simulink model "martins_version_wconv"  (R2023b)
settings: Solver=VariableStepAuto  StartTime=0.0  StopTime=Tend  RelTol=1e-3
undefined symbols (not defined in the file): C_dc, c_f, C_hv_km, Cagg, DiscIntNeverNeededParam, H_vsm, Ibase_hv, Ibase_lv, Ibase_mv, k_AD, k_d_vsm, k_decouple, k_ffv, k_ic, k_idc, k_mod, k_p_p_vsm, k_p_q_vsm, k_pc, k_pdc, k_vc, KG_LL, ki, KI_LL, ki_q, kp, KP_LL, kslope_VSC, L_comp, l_f, l_f_si1, l_grid, L_hv_km, l_t_ehvhv, l_t_hvmv, l_t_mvlv, L_Virt, Lagg, Lbase1v, length_export, omega_nom, P_aero_0, phase_shift_test_state, phase_shifts, pie_export, r_f, r_f_si1, r_grid, R_hv_km, r_t_ehvhv, r_t_hvmv, r_t_mvlv, R_Virt, Ragg, rocof_slope, Rocof_test_state, Sbase1, Tchange_gfm_ref, Tdelay, Trocof_end ... (+13)
libraries: slpidlib x11, spsFirstOrderFilterLib x3, cstblocks x1, simulink x1, spsSampleandHoldLib x1, spspowerguiLib x1
(part 3 of 3)

== system martins_version_wconv/GFC_WT/grid>>PLL2 ==
  note: *
  note: =
  note: inv ([  cos(wt)   sin(wt)
      |    -sin(wt)    cos(wt)   ])
  note: [ d
      |    q ]
  note: [  al
      |     be  ]
  note: *
  note: =
  note: [  cos(wt)   -sin(wt)
      |    sin(wt)    cos(wt)   ]
  note: [ d
      |    q ]
  note: [  al
      |     be  ]
  vgDQ : Inport
  wt : Inport  Port=2
  Cos : Trigonometry  Operator=cos
  Demux1 : Demux  Outputs=2
  Display5 : Display
  Mux3 : Mux  Inputs=2
  Product{,1..3} (4 alike) : Product
  Sin : Trigonometry
  Sum : Sum
  Sum1 : Sum  Inputs=+-
  vgdq : Outport  InitialOutput=[0,0]  VectorParamsAs1DForOutWhenUnconnected=off
  wires:
  Demux1/1 -> Product/1, Product3/1
  wt/1 -> Sin/1, Cos/1
  Product/1 -> Sum/1
  Sum/1 -> Mux3/1
  Mux3/1 -> Display5/1, vgdq/1
  Sum1/1 -> Mux3/2
  vgDQ/1 -> Demux1/1
  Sin/1 -> Product1/2, Product3/2
  Product1/1 -> Sum/2
  Cos/1 -> Product/2, Product2/2
  Product2/1 -> Sum1/1
  Demux1/2 -> Product1/1, Product2/1
  Product3/1 -> Sum1/2

== system martins_version_wconv/GFC_WT/grid>>PLL3 ==
  note: *
  note: =
  note: inv ([  cos(wt)   sin(wt)
      |    -sin(wt)    cos(wt)   ])
  note: [ d
      |    q ]
  note: [  al
      |     be  ]
  note: *
  note: =
  note: [  cos(wt)   -sin(wt)
      |    sin(wt)    cos(wt)   ]
  note: [ d
      |    q ]
  note: [  al
      |     be  ]
  vgDQ : Inport
  wt : Inport  Port=2
  Cos : Trigonometry  Operator=cos
  Demux1 : Demux  Outputs=2
  Display5 : Display
  Mux3 : Mux  Inputs=[vect vect]
  Product{,1..3} (4 alike) : Product
  Sin : Trigonometry
  Sum : Sum
  Sum1 : Sum  Inputs=+-
  vgdq : Outport  InitialOutput=[0,0]  VectorParamsAs1DForOutWhenUnconnected=off
  wires:
  Demux1/1 -> Product/1, Product3/1
  wt/1 -> Sin/1, Cos/1
  Product/1 -> Sum/1
  Sum/1 -> Mux3/1
  Mux3/1 -> Display5/1, vgdq/1
  Sum1/1 -> Mux3/2
  vgDQ/1 -> Demux1/1
  Sin/1 -> Product1/2, Product3/2
  Product1/1 -> Sum/2
  Cos/1 -> Product/2, Product2/2
  Product2/1 -> Sum1/1
  Demux1/2 -> Product1/1, Product2/1
  Product3/1 -> Sum1/2

== system martins_version_wconv/GFC_WT/v_dc_reg ==
  In1 : Inport
  Ipart : DiscreteIntegrator  Commented=on  gainval=k_idc  SampleTime=-1  ICPrevOutput=DiscIntNeverNeededParam  ICPrevScaledInput=DiscIntNeverNeededParam
  PID Controller : slpidlib/PID Controller  Controller=PI  Form=Parallel  TimeDomain=Continuous-time  UseExternalTs=off  SampleTime=-1  IntegratorMethod=Forward Euler  FilterMethod=Forward Euler  ControllerParametersSource=internal  P=k_pdc  I=k_idc  UseKiTs=off  D=0  N=100  UseFilter=on  TunerSelectOption=Transfer Function Based (PID Tuner App)  InitialConditionSource=internal  InitialConditionForIntegrator=0  InitialConditionForFilter=0  DifferentiatorICPrevScaledInput=0  ExternalReset=none  TrackingMode=off  Kt=1  LimitOutput=off  SatLimitsSource=internal  UpperSaturationLimit=inf  LowerSaturationLimit=-inf  LinearizeAsGain=on  AntiWindupMode=none  Kb=1  LimitIntegrator=off  UpperIntegratorSaturationLimit=inf  LowerIntegratorSaturationLimit=-inf  POutMin=[]  POutMax=[]  IOutMin=[]  IOutMax=[]  DOutMin=[]  DOutMax=[]  NOutMin=[]  NOutMax=[]  SumOutMin=[]  SumOutMax=[]  SaturationOutMin=[]  SaturationOutMax=[]  PParamMin=[]  PParamMax=[]  IParamMin=[]  IParamMax=[]  DParamMin=[]  DParamMax=[]  NParamMin=[]  NParamMax=[]  KbParamMin=[]  KbParamMax=[]  KtParamMin=[]  KtParamMax=[]  KbOutMin=[]  KbOutMax=[]  KtOutMin=[]  KtOutMax=[]  IntegratorOutMin=[]  IntegratorOutMax=[]  FilterOutMin=[]  FilterOutMax=[]  SumI1OutMin=[]  SumI1OutMax=[]  SumI2OutMin=[]  SumI2OutMax=[]  SumI3OutMin=[]  SumI3OutMax=[]  SumI4OutMin=[]  SumI4OutMax=[]  SumDOutMin=[]  SumDOutMax=[]  DifferentiatorOutMin=[]  DifferentiatorOutMax=[]  FilterDiffOutCoefMin=[]  FilterDiffOutCoefMax=[]  ReciprocalOutMin=[]  ReciprocalOutMax=[]  SumDenOutMin=[]  SumDenOutMax=[]  SumNumOutMin=[]  SumNumOutMax=[]  DivideOutMin=[]  DivideOutMax=[]  UdiffTsProdOutMin=[]  UdiffTsProdOutMax=[]  NTsProdOutMin=[]  NTsProdOutMax=[]  UintegralTsProdOutMin=[]  UintegralTsProdOutMax=[]  UngainTsProdOutMin=[]  UngainTsProdOutMax=[]  ClampingZeroOutDataTypeStr=Inherit: Inherit via back propagation  ClampingZeroOutMin=[]  ClampingZeroOutMax=[]  FilterDenConstantOutDataTypeStr=Inherit: Inherit via back propagation  FilterDenConstantOutMin=[]  FilterDenConstantOutMax=[]  PCopyOutDataTypeStr=Inherit: Inherit via back propagation  PCopyOutMin=[]  PCopyOutMax=[]  NCopyOutDataTypeStr=Inherit: Inherit via back propagation  NCopyOutMin=[]  NCopyOutMax=[]  IntegratorContinuousStateAttributes=''  IntegratorStateMustResolveToSignalObject=off  IntegratorRTWStateStorageClass=Auto  FilterContinuousStateAttributes=''  FilterStateMustResolveToSignalObject=off  FilterRTWStateStorageClass=Auto  ParallelPVariant=InternalParameters  IdealPVariant=Disabled  IVariant=InternalParameters  DVariant=Disabled  IntegratorVariant=Continuous  SatVariant=Disabled  AWVariant=Passthrough  PCopyVariant=Disabled  TRVariant=Disabled  FdbkBlocksVariant=Forward  IdealPFdbkVariant=Disabled  SatFdbkVariant=Disabled  DerivativeFilterVariant=Disabled  NVariant=Disabled  NCopyVariant=Disabled_SignalSpec  FilterICVariant=Disabled  IntegratorICVariant=InternalICs  ExternalResetVariant=Disabled  TRSumVariant=Passthrough  SumFdbkVariant=Disabled  SumVariant=Sum_PI  TsampFilterVariant=InternalTs  TsampNgainVariant=Passthrough  TsampIntegralVariant=Disabled_SignalSpec  ExternalSaturationOutDataTypeStr=Inherit: Same as second input
  Ppart : Gain  Commented=on  Gain=k_pdc  SaturateOnIntegerOverflow=on  OutDataTypeStr=Inherit: Same as input  ParamDataTypeStr=Inherit: Same as input
  Sum5 : Sum  Commented=on  Inputs=|++  InputSameDT=on  SaturateOnIntegerOverflow=on  OutDataTypeStr=Inherit: Same as first input
  W : Outport
  wires:
  Ppart/1 -> Sum5/1
  Ipart/1 -> Sum5/2
  In1/1 -> PID Controller/1, Ppart/1, Ipart/1
  PID Controller/1 -> W/1

== system martins_version_wconv/HVAC CABLE 10 PI SEGMENTS 1/RC sys1 ==
  note: Left shunt capacitor
  note: shunt capacitor
  Iload_DQ : Inport
  "Isource_DQ " : Inport  Port=2
  omega_ref : Inport  Port=3
  1 : Gain  Gain=Rd
  10 : Gain  Gain=inv_Csource
  2 : Gain  Gain=Rd
  8 : Gain  Gain=Csource
  9 : Gain  Gain=inv_Csource
  Demux2 : Demux  Outputs=2
  Demux3 : Demux  Outputs=2
  Display1 : Display
  Display6 : Display
  Mux1 : Mux  Inputs=2
  Mux2 : Mux  Inputs=2
  Product7 : Product
  Product8 : Product
  Sum1 : Sum  Inputs=|++
  Sum14 : Sum  Inputs=|+--
  Sum15 : Sum  Inputs=|++-
  Sum2 : Sum  Inputs=|++
  Sum3 : Sum  Inputs=|+-
  Sum4 : Sum  Inputs=|+-
  Vcd : Scope
  VcpdR_int : Integrator  InitialCondition=VD0  UpperSaturationLimit=50  LowerSaturationLimit=-1000
  VcpqR_int : Integrator  InitialCondition=VQ0  UpperSaturationLimit=50  LowerSaturationLimit=-1000
  Vcq : Scope
  VpccR_DQ : Outport  VectorParamsAs1DForOutWhenUnconnected=off
  wires:
  8/1 -> [wcs], Display1/1
  Mux1/1 -> VpccR_DQ/1
  Product8/1 -> Sum14/3
  Sum15/1 -> 9/1
  10/1 -> VcpqR_int/1
  Product7/1 -> Sum15/1
  VcpqR_int/1 -> Mux2/1, Sum2/1, Product7/2, Vcq/1
  [wcs] -> Product7/1, Product8/1
  Sum14/1 -> 10/1
  9/1 -> VcpdR_int/1
  omega_ref/1 -> 8/1
  Demux2/1 -> Sum4/1, Sum15/2
  Demux2/2 -> Sum3/1, Sum14/1
  Iload_DQ/1 -> Demux2/1
  "Isource_DQ "/1 -> Demux3/1
  Demux3/2 -> Sum3/2, Sum14/2
  Demux3/1 -> Sum4/2, Sum15/3
  VcpdR_int/1 -> Mux2/2, Product8/2, Sum1/1
  Sum1/1 -> Mux1/1
  Sum2/1 -> Mux1/2
  1/1 -> Sum2/2
  2/1 -> Sum1/2
  Mux2/1 -> Display6/1
  Sum3/1 -> 1/1
  Sum4/1 -> 2/1

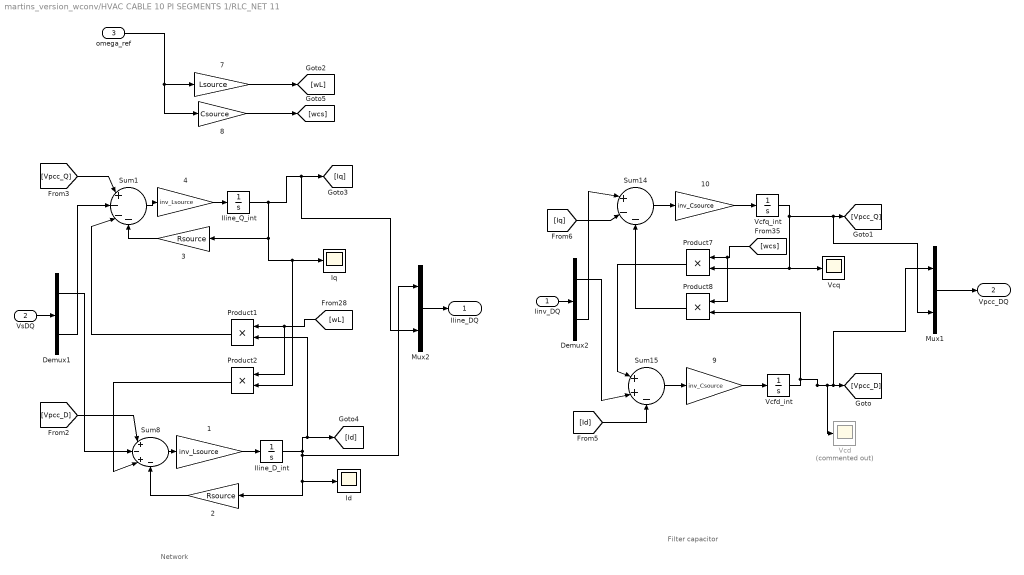
== system martins_version_wconv/HVAC CABLE 10 PI SEGMENTS 1/RLC_NET 11 ==
  note: Network
  note: Filter capacitor
  Iinv_DQ : Inport
  "VsDQ " : Inport  Port=2
  omega_ref : Inport  Port=3
  1 : Gain  Gain=inv_Lsource
  10 : Gain  Gain=inv_Csource
  2 : Gain  Gain=Rsource
  3 : Gain  Gain=Rsource
  4 : Gain  Gain=inv_Lsource
  7 : Gain  Gain=Lsource
  8 : Gain  Gain=Csource
  9 : Gain  Gain=inv_Csource
  Demux1 : Demux  Outputs=2
  Demux2 : Demux  Outputs=2
  Id : Scope
  Iline_D_int : Integrator  UpperSaturationLimit=50  LowerSaturationLimit=-1000
  Iline_Q_int : Integrator  UpperSaturationLimit=50  LowerSaturationLimit=-1000
  Iq : Scope
  Mux1 : Mux  Inputs=2
  Mux2 : Mux  Inputs=2
  Product{1..2,7..8} (4 alike) : Product
  Sum1 : Sum  Inputs=|+---
  Sum14 : Sum  Inputs=|+--
  Sum15 : Sum  Inputs=|++-
  Sum8 : Sum  Inputs=|+-+-
  Vcd : Scope  Commented=on
  Vcfd_int : Integrator  UpperSaturationLimit=50  LowerSaturationLimit=-1000
  Vcfq_int : Integrator  UpperSaturationLimit=50  LowerSaturationLimit=-1000
  Vcq : Scope
  Iline_DQ : Outport  VectorParamsAs1DForOutWhenUnconnected=off
  Vpcc_DQ : Outport  Port=2  VectorParamsAs1DForOutWhenUnconnected=off
  wires:
  Mux2/1 -> Iline_DQ/1
  Iinv_DQ/1 -> Demux2/1
  Demux2/2 -> Sum14/1
  Demux2/1 -> Sum15/2
  [wL] -> Product2/1, Product1/1
  Product1/1 -> Sum1/3
  4/1 -> Iline_Q_int/1
  3/1 -> Sum1/4
  Product2/1 -> Sum8/3
  2/1 -> Sum8/4
  Sum8/1 -> 1/1
  Iline_Q_int/1 -> 3/1, Product2/2, Iq/1, [Iq], Mux2/2
  Iline_D_int/1 -> Mux2/1, 2/1, Id/1, Product1/2, [Id]
  1/1 -> Iline_D_int/1
  Sum1/1 -> 4/1
  [Vpcc_D] -> Sum8/1
  [Vpcc_Q] -> Sum1/1
  omega_ref/1 -> 8/1, 7/1
  7/1 -> [wL]
  9/1 -> Vcfd_int/1
  Sum14/1 -> 10/1
  [wcs] -> Product8/1, Product7/1
  [Id] -> Sum15/3
  Vcfq_int/1 -> Mux1/2, [Vpcc_Q], Product7/2, Vcq/1
  Product7/1 -> Sum15/1
  [Iq] -> Sum14/2
  10/1 -> Vcfq_int/1
  Sum15/1 -> 9/1
  Product8/1 -> Sum14/3
  8/1 -> [wcs]
  Vcfd_int/1 -> Product8/2, Mux1/1, [Vpcc_D], Vcd/1
  Mux1/1 -> Vpcc_DQ/1
  Demux1/1 -> Sum8/2
  Demux1/2 -> Sum1/2
  "VsDQ "/1 -> Demux1/1

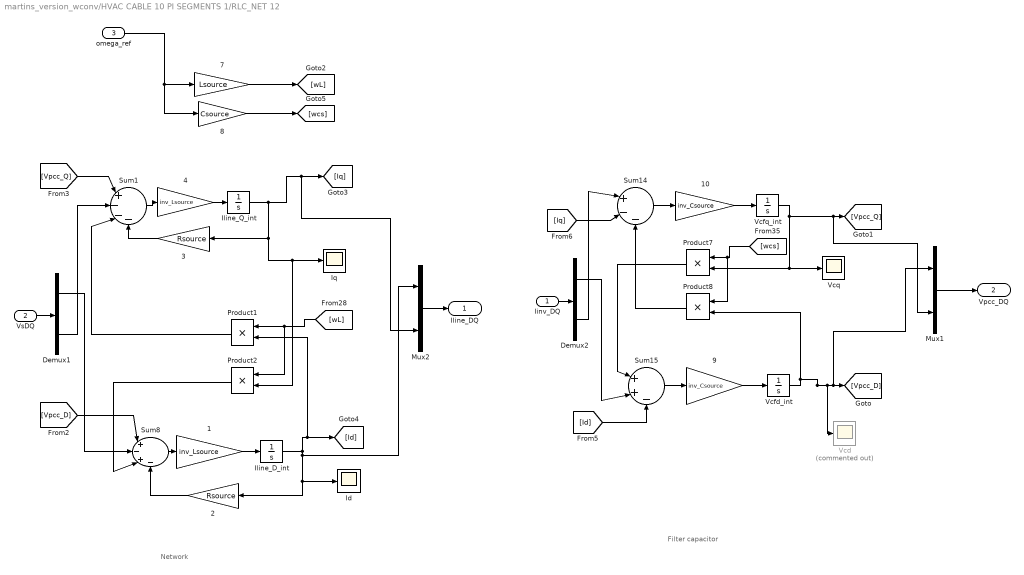
== system martins_version_wconv/HVAC CABLE 10 PI SEGMENTS 1/RLC_NET 12 ==
  note: Filter capacitor
  note: Network
  Iinv_DQ : Inport
  "VsDQ " : Inport  Port=2
  omega_ref : Inport  Port=3
  1 : Gain  Gain=inv_Lsource
  10 : Gain  Gain=inv_Csource
  2 : Gain  Gain=Rsource
  3 : Gain  Gain=Rsource
  4 : Gain  Gain=inv_Lsource
  7 : Gain  Gain=Lsource
  8 : Gain  Gain=Csource
  9 : Gain  Gain=inv_Csource
  Demux1 : Demux  Outputs=2
  Demux2 : Demux  Outputs=2
  Id : Scope
  Iline_D_int : Integrator  UpperSaturationLimit=50  LowerSaturationLimit=-1000
  Iline_Q_int : Integrator  UpperSaturationLimit=50  LowerSaturationLimit=-1000
  Iq : Scope
  Mux1 : Mux  Inputs=2
  Mux2 : Mux  Inputs=2
  Product{1..2,7..8} (4 alike) : Product
  Sum1 : Sum  Inputs=|+---
  Sum14 : Sum  Inputs=|+--
  Sum15 : Sum  Inputs=|++-
  Sum8 : Sum  Inputs=|+-+-
  Vcd : Scope  Commented=on
  Vcfd_int : Integrator  UpperSaturationLimit=50  LowerSaturationLimit=-1000
  Vcfq_int : Integrator  UpperSaturationLimit=50  LowerSaturationLimit=-1000
  Vcq : Scope
  Iline_DQ : Outport  VectorParamsAs1DForOutWhenUnconnected=off
  Vpcc_DQ : Outport  Port=2  VectorParamsAs1DForOutWhenUnconnected=off
  wires:
  "VsDQ "/1 -> Demux1/1
  Demux1/2 -> Sum1/2
  Demux1/1 -> Sum8/2
  Mux1/1 -> Vpcc_DQ/1
  Vcfd_int/1 -> Vcd/1, [Vpcc_D], Mux1/1, Product8/2
  8/1 -> [wcs]
  Product8/1 -> Sum14/3
  Sum15/1 -> 9/1
  10/1 -> Vcfq_int/1
  [Iq] -> Sum14/2
  Product7/1 -> Sum15/1
  Vcfq_int/1 -> Vcq/1, Product7/2, [Vpcc_Q], Mux1/2
  [Id] -> Sum15/3
  [wcs] -> Product7/1, Product8/1
  Sum14/1 -> 10/1
  9/1 -> Vcfd_int/1
  7/1 -> [wL]
  omega_ref/1 -> 7/1, 8/1
  [Vpcc_Q] -> Sum1/1
  [Vpcc_D] -> Sum8/1
  Sum1/1 -> 4/1
  1/1 -> Iline_D_int/1
  Iline_D_int/1 -> [Id], Product1/2, Id/1, 2/1, Mux2/1
  Iline_Q_int/1 -> Mux2/2, [Iq], Iq/1, Product2/2, 3/1
  Sum8/1 -> 1/1
  2/1 -> Sum8/4
  Product2/1 -> Sum8/3
  3/1 -> Sum1/4
  4/1 -> Iline_Q_int/1
  Product1/1 -> Sum1/3
  [wL] -> Product1/1, Product2/1
  Demux2/1 -> Sum15/2
  Demux2/2 -> Sum14/1
  Iinv_DQ/1 -> Demux2/1
  Mux2/1 -> Iline_DQ/1

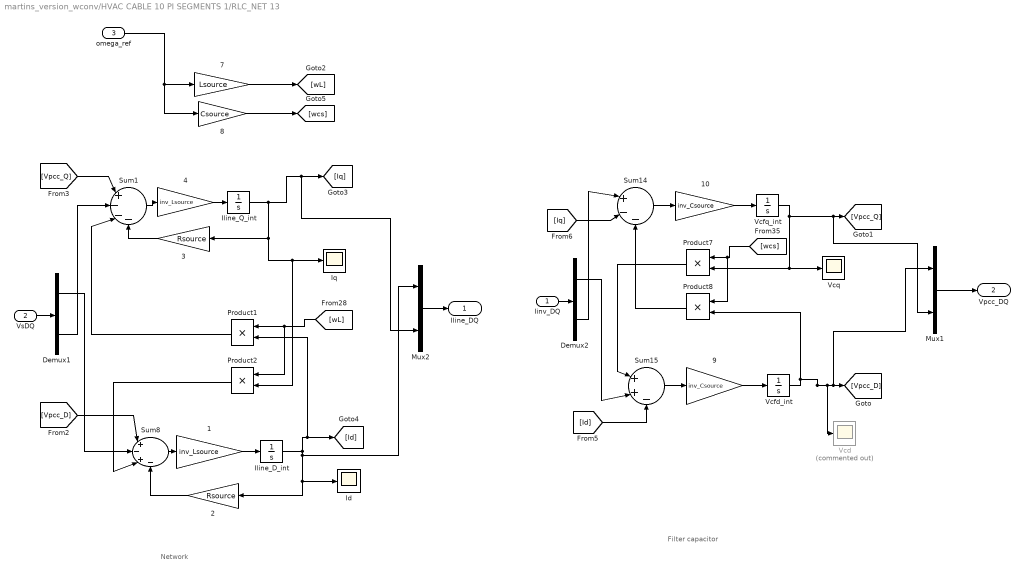
== system martins_version_wconv/HVAC CABLE 10 PI SEGMENTS 1/RLC_NET 13 ==
  note: Filter capacitor
  note: Network
  Iinv_DQ : Inport
  "VsDQ " : Inport  Port=2
  omega_ref : Inport  Port=3
  1 : Gain  Gain=inv_Lsource
  10 : Gain  Gain=inv_Csource
  2 : Gain  Gain=Rsource
  3 : Gain  Gain=Rsource
  4 : Gain  Gain=inv_Lsource
  7 : Gain  Gain=Lsource
  8 : Gain  Gain=Csource
  9 : Gain  Gain=inv_Csource
  Demux1 : Demux  Outputs=2
  Demux2 : Demux  Outputs=2
  Id : Scope
  Iline_D_int : Integrator  UpperSaturationLimit=50  LowerSaturationLimit=-1000
  Iline_Q_int : Integrator  UpperSaturationLimit=50  LowerSaturationLimit=-1000
  Iq : Scope
  Mux1 : Mux  Inputs=2
  Mux2 : Mux  Inputs=2
  Product{1..2,7..8} (4 alike) : Product
  Sum1 : Sum  Inputs=|+---
  Sum14 : Sum  Inputs=|+--
  Sum15 : Sum  Inputs=|++-
  Sum8 : Sum  Inputs=|+-+-
  Vcd : Scope  Commented=on
  Vcfd_int : Integrator  UpperSaturationLimit=50  LowerSaturationLimit=-1000
  Vcfq_int : Integrator  UpperSaturationLimit=50  LowerSaturationLimit=-1000
  Vcq : Scope
  Iline_DQ : Outport  VectorParamsAs1DForOutWhenUnconnected=off
  Vpcc_DQ : Outport  Port=2  VectorParamsAs1DForOutWhenUnconnected=off
  wires:
  "VsDQ "/1 -> Demux1/1
  Demux1/2 -> Sum1/2
  Demux1/1 -> Sum8/2
  Mux1/1 -> Vpcc_DQ/1
  Vcfd_int/1 -> Vcd/1, [Vpcc_D], Mux1/1, Product8/2
  8/1 -> [wcs]
  Product8/1 -> Sum14/3
  Sum15/1 -> 9/1
  10/1 -> Vcfq_int/1
  [Iq] -> Sum14/2
  Product7/1 -> Sum15/1
  Vcfq_int/1 -> Vcq/1, Product7/2, [Vpcc_Q], Mux1/2
  [Id] -> Sum15/3
  [wcs] -> Product7/1, Product8/1
  Sum14/1 -> 10/1
  9/1 -> Vcfd_int/1
  7/1 -> [wL]
  omega_ref/1 -> 7/1, 8/1
  [Vpcc_Q] -> Sum1/1
  [Vpcc_D] -> Sum8/1
  Sum1/1 -> 4/1
  1/1 -> Iline_D_int/1
  Iline_D_int/1 -> [Id], Product1/2, Id/1, 2/1, Mux2/1
  Iline_Q_int/1 -> Mux2/2, [Iq], Iq/1, Product2/2, 3/1
  Sum8/1 -> 1/1
  2/1 -> Sum8/4
  Product2/1 -> Sum8/3
  3/1 -> Sum1/4
  4/1 -> Iline_Q_int/1
  Product1/1 -> Sum1/3
  [wL] -> Product1/1, Product2/1
  Demux2/1 -> Sum15/2
  Demux2/2 -> Sum14/1
  Iinv_DQ/1 -> Demux2/1
  Mux2/1 -> Iline_DQ/1

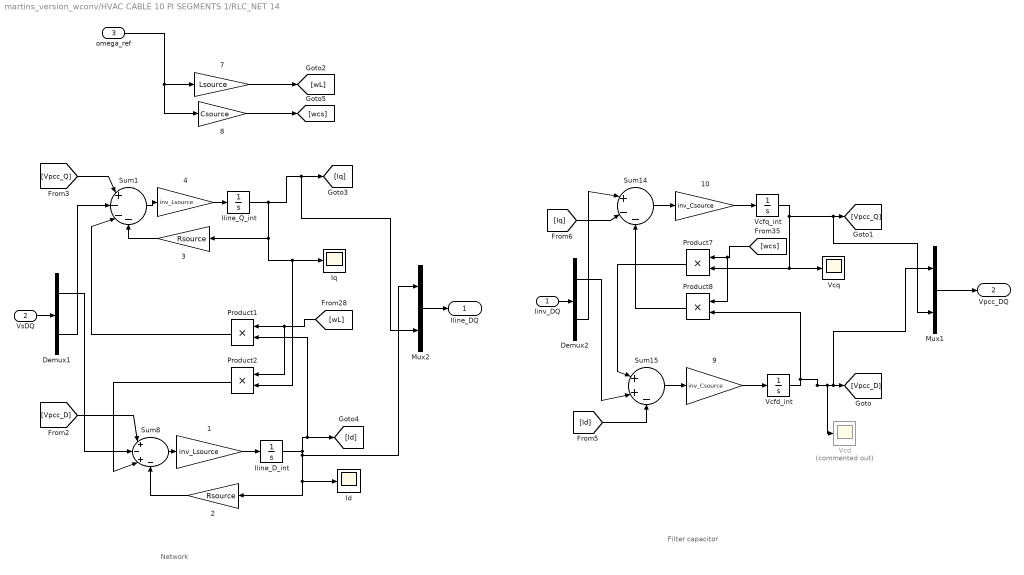
== system martins_version_wconv/HVAC CABLE 10 PI SEGMENTS 1/RLC_NET 14 ==
  note: Network
  note: Filter capacitor
  Iinv_DQ : Inport
  "VsDQ " : Inport  Port=2
  omega_ref : Inport  Port=3
  1 : Gain  Gain=inv_Lsource
  10 : Gain  Gain=inv_Csource
  2 : Gain  Gain=Rsource
  3 : Gain  Gain=Rsource
  4 : Gain  Gain=inv_Lsource
  7 : Gain  Gain=Lsource
  8 : Gain  Gain=Csource
  9 : Gain  Gain=inv_Csource
  Demux1 : Demux  Outputs=2
  Demux2 : Demux  Outputs=2
  Id : Scope
  Iline_D_int : Integrator  UpperSaturationLimit=50  LowerSaturationLimit=-1000
  Iline_Q_int : Integrator  UpperSaturationLimit=50  LowerSaturationLimit=-1000
  Iq : Scope
  Mux1 : Mux  Inputs=2
  Mux2 : Mux  Inputs=2
  Product{1..2,7..8} (4 alike) : Product
  Sum1 : Sum  Inputs=|+---
  Sum14 : Sum  Inputs=|+--
  Sum15 : Sum  Inputs=|++-
  Sum8 : Sum  Inputs=|+-+-
  Vcd : Scope  Commented=on
  Vcfd_int : Integrator  UpperSaturationLimit=50  LowerSaturationLimit=-1000
  Vcfq_int : Integrator  UpperSaturationLimit=50  LowerSaturationLimit=-1000
  Vcq : Scope
  Iline_DQ : Outport  VectorParamsAs1DForOutWhenUnconnected=off
  Vpcc_DQ : Outport  Port=2  VectorParamsAs1DForOutWhenUnconnected=off
  wires:
  Mux2/1 -> Iline_DQ/1
  Iinv_DQ/1 -> Demux2/1
  Demux2/2 -> Sum14/1
  Demux2/1 -> Sum15/2
  [wL] -> Product2/1, Product1/1
  Product1/1 -> Sum1/3
  4/1 -> Iline_Q_int/1
  3/1 -> Sum1/4
  Product2/1 -> Sum8/3
  2/1 -> Sum8/4
  Sum8/1 -> 1/1
  Iline_Q_int/1 -> 3/1, Product2/2, Iq/1, [Iq], Mux2/2
  Iline_D_int/1 -> Mux2/1, 2/1, Id/1, Product1/2, [Id]
  1/1 -> Iline_D_int/1
  Sum1/1 -> 4/1
  [Vpcc_D] -> Sum8/1
  [Vpcc_Q] -> Sum1/1
  omega_ref/1 -> 8/1, 7/1
  7/1 -> [wL]
  9/1 -> Vcfd_int/1
  Sum14/1 -> 10/1
  [wcs] -> Product8/1, Product7/1
  [Id] -> Sum15/3
  Vcfq_int/1 -> Mux1/2, [Vpcc_Q], Product7/2, Vcq/1
  Product7/1 -> Sum15/1
  [Iq] -> Sum14/2
  10/1 -> Vcfq_int/1
  Sum15/1 -> 9/1
  Product8/1 -> Sum14/3
  8/1 -> [wcs]
  Vcfd_int/1 -> Product8/2, Mux1/1, [Vpcc_D], Vcd/1
  Mux1/1 -> Vpcc_DQ/1
  Demux1/1 -> Sum8/2
  Demux1/2 -> Sum1/2
  "VsDQ "/1 -> Demux1/1

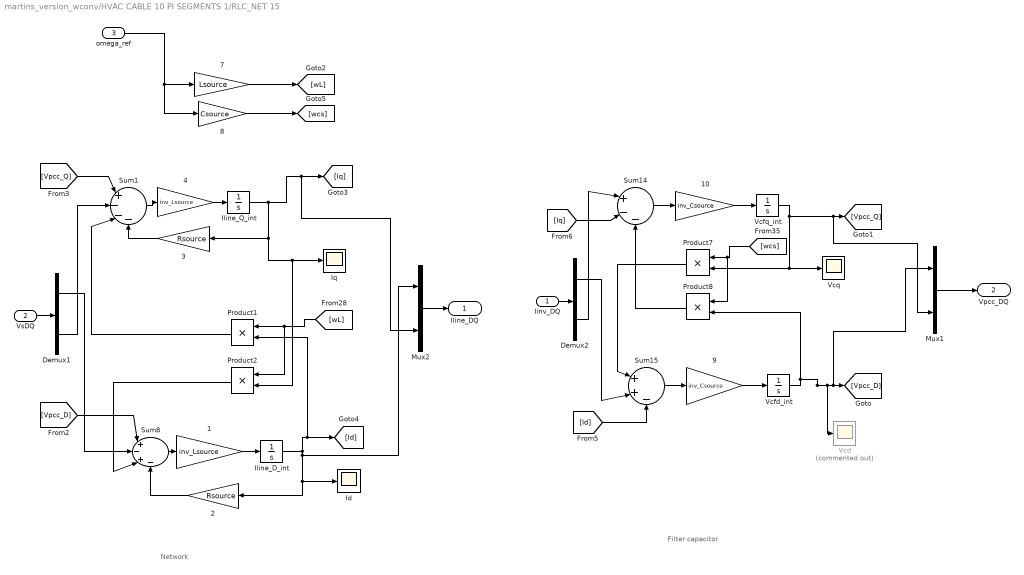
== system martins_version_wconv/HVAC CABLE 10 PI SEGMENTS 1/RLC_NET 15 ==
  note: Filter capacitor
  note: Network
  Iinv_DQ : Inport
  "VsDQ " : Inport  Port=2
  omega_ref : Inport  Port=3
  1 : Gain  Gain=inv_Lsource
  10 : Gain  Gain=inv_Csource
  2 : Gain  Gain=Rsource
  3 : Gain  Gain=Rsource
  4 : Gain  Gain=inv_Lsource
  7 : Gain  Gain=Lsource
  8 : Gain  Gain=Csource
  9 : Gain  Gain=inv_Csource
  Demux1 : Demux  Outputs=2
  Demux2 : Demux  Outputs=2
  Id : Scope
  Iline_D_int : Integrator  UpperSaturationLimit=50  LowerSaturationLimit=-1000
  Iline_Q_int : Integrator  UpperSaturationLimit=50  LowerSaturationLimit=-1000
  Iq : Scope
  Mux1 : Mux  Inputs=2
  Mux2 : Mux  Inputs=2
  Product{1..2,7..8} (4 alike) : Product
  Sum1 : Sum  Inputs=|+---
  Sum14 : Sum  Inputs=|+--
  Sum15 : Sum  Inputs=|++-
  Sum8 : Sum  Inputs=|+-+-
  Vcd : Scope  Commented=on
  Vcfd_int : Integrator  UpperSaturationLimit=50  LowerSaturationLimit=-1000
  Vcfq_int : Integrator  UpperSaturationLimit=50  LowerSaturationLimit=-1000
  Vcq : Scope
  Iline_DQ : Outport  VectorParamsAs1DForOutWhenUnconnected=off
  Vpcc_DQ : Outport  Port=2  VectorParamsAs1DForOutWhenUnconnected=off
  wires:
  "VsDQ "/1 -> Demux1/1
  Demux1/2 -> Sum1/2
  Demux1/1 -> Sum8/2
  Mux1/1 -> Vpcc_DQ/1
  Vcfd_int/1 -> Vcd/1, [Vpcc_D], Mux1/1, Product8/2
  8/1 -> [wcs]
  Product8/1 -> Sum14/3
  Sum15/1 -> 9/1
  10/1 -> Vcfq_int/1
  [Iq] -> Sum14/2
  Product7/1 -> Sum15/1
  Vcfq_int/1 -> Vcq/1, Product7/2, [Vpcc_Q], Mux1/2
  [Id] -> Sum15/3
  [wcs] -> Product7/1, Product8/1
  Sum14/1 -> 10/1
  9/1 -> Vcfd_int/1
  7/1 -> [wL]
  omega_ref/1 -> 7/1, 8/1
  [Vpcc_Q] -> Sum1/1
  [Vpcc_D] -> Sum8/1
  Sum1/1 -> 4/1
  1/1 -> Iline_D_int/1
  Iline_D_int/1 -> [Id], Product1/2, Id/1, 2/1, Mux2/1
  Iline_Q_int/1 -> Mux2/2, [Iq], Iq/1, Product2/2, 3/1
  Sum8/1 -> 1/1
  2/1 -> Sum8/4
  Product2/1 -> Sum8/3
  3/1 -> Sum1/4
  4/1 -> Iline_Q_int/1
  Product1/1 -> Sum1/3
  [wL] -> Product1/1, Product2/1
  Demux2/1 -> Sum15/2
  Demux2/2 -> Sum14/1
  Iinv_DQ/1 -> Demux2/1
  Mux2/1 -> Iline_DQ/1

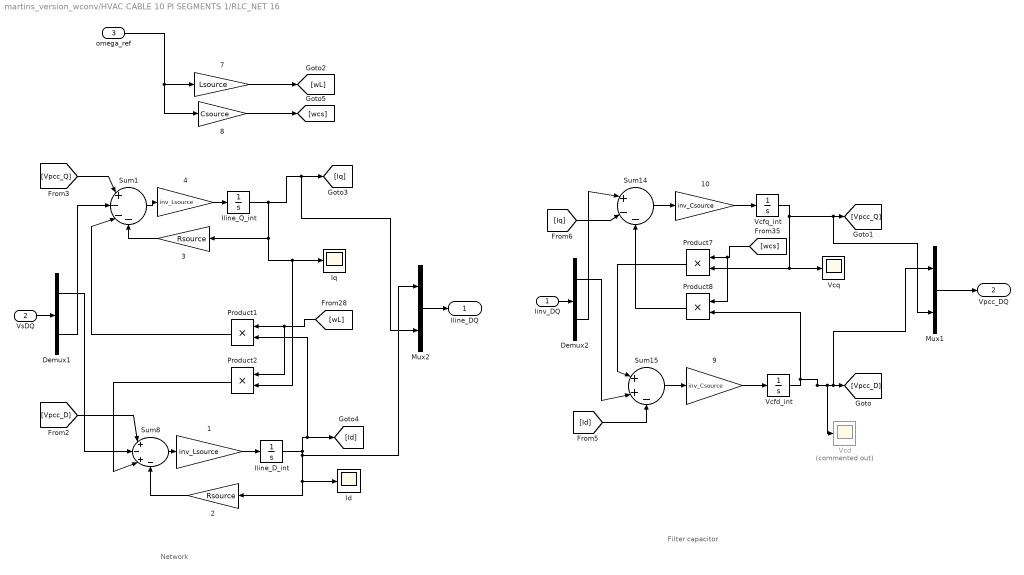
== system martins_version_wconv/HVAC CABLE 10 PI SEGMENTS 1/RLC_NET 16 ==
  note: Filter capacitor
  note: Network
  Iinv_DQ : Inport
  "VsDQ " : Inport  Port=2
  omega_ref : Inport  Port=3
  1 : Gain  Gain=inv_Lsource
  10 : Gain  Gain=inv_Csource
  2 : Gain  Gain=Rsource
  3 : Gain  Gain=Rsource
  4 : Gain  Gain=inv_Lsource
  7 : Gain  Gain=Lsource
  8 : Gain  Gain=Csource
  9 : Gain  Gain=inv_Csource
  Demux1 : Demux  Outputs=2
  Demux2 : Demux  Outputs=2
  Id : Scope
  Iline_D_int : Integrator  UpperSaturationLimit=50  LowerSaturationLimit=-1000
  Iline_Q_int : Integrator  UpperSaturationLimit=50  LowerSaturationLimit=-1000
  Iq : Scope
  Mux1 : Mux  Inputs=2
  Mux2 : Mux  Inputs=2
  Product{1..2,7..8} (4 alike) : Product
  Sum1 : Sum  Inputs=|+---
  Sum14 : Sum  Inputs=|+--
  Sum15 : Sum  Inputs=|++-
  Sum8 : Sum  Inputs=|+-+-
  Vcd : Scope  Commented=on
  Vcfd_int : Integrator  UpperSaturationLimit=50  LowerSaturationLimit=-1000
  Vcfq_int : Integrator  UpperSaturationLimit=50  LowerSaturationLimit=-1000
  Vcq : Scope
  Iline_DQ : Outport  VectorParamsAs1DForOutWhenUnconnected=off
  Vpcc_DQ : Outport  Port=2  VectorParamsAs1DForOutWhenUnconnected=off
  wires:
  "VsDQ "/1 -> Demux1/1
  Demux1/2 -> Sum1/2
  Demux1/1 -> Sum8/2
  Mux1/1 -> Vpcc_DQ/1
  Vcfd_int/1 -> Vcd/1, [Vpcc_D], Mux1/1, Product8/2
  8/1 -> [wcs]
  Product8/1 -> Sum14/3
  Sum15/1 -> 9/1
  10/1 -> Vcfq_int/1
  [Iq] -> Sum14/2
  Product7/1 -> Sum15/1
  Vcfq_int/1 -> Vcq/1, Product7/2, [Vpcc_Q], Mux1/2
  [Id] -> Sum15/3
  [wcs] -> Product7/1, Product8/1
  Sum14/1 -> 10/1
  9/1 -> Vcfd_int/1
  7/1 -> [wL]
  omega_ref/1 -> 7/1, 8/1
  [Vpcc_Q] -> Sum1/1
  [Vpcc_D] -> Sum8/1
  Sum1/1 -> 4/1
  1/1 -> Iline_D_int/1
  Iline_D_int/1 -> [Id], Product1/2, Id/1, 2/1, Mux2/1
  Iline_Q_int/1 -> Mux2/2, [Iq], Iq/1, Product2/2, 3/1
  Sum8/1 -> 1/1
  2/1 -> Sum8/4
  Product2/1 -> Sum8/3
  3/1 -> Sum1/4
  4/1 -> Iline_Q_int/1
  Product1/1 -> Sum1/3
  [wL] -> Product1/1, Product2/1
  Demux2/1 -> Sum15/2
  Demux2/2 -> Sum14/1
  Iinv_DQ/1 -> Demux2/1
  Mux2/1 -> Iline_DQ/1

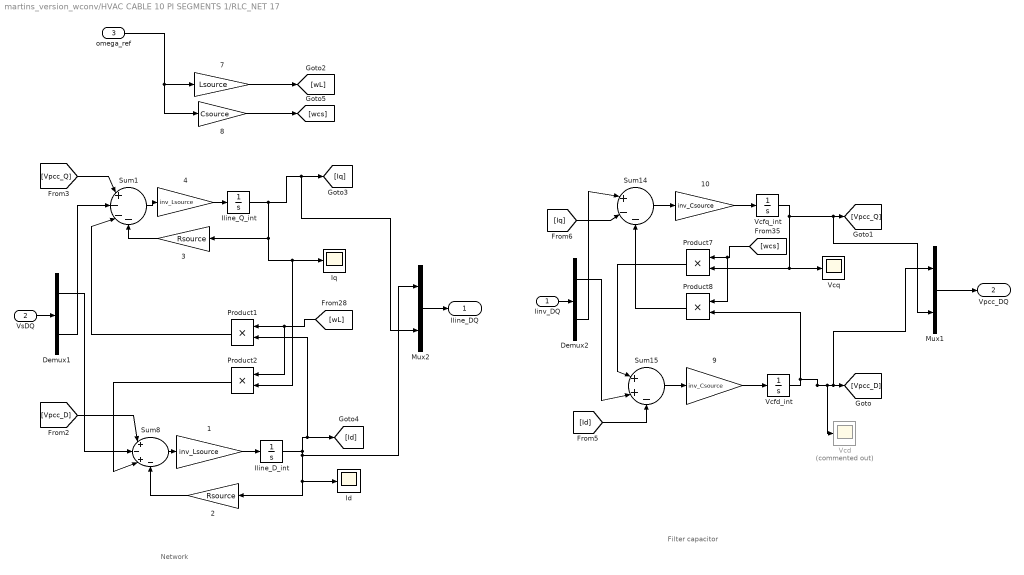
== system martins_version_wconv/HVAC CABLE 10 PI SEGMENTS 1/RLC_NET 17 ==
  note: Network
  note: Filter capacitor
  Iinv_DQ : Inport
  "VsDQ " : Inport  Port=2
  omega_ref : Inport  Port=3
  1 : Gain  Gain=inv_Lsource
  10 : Gain  Gain=inv_Csource
  2 : Gain  Gain=Rsource
  3 : Gain  Gain=Rsource
  4 : Gain  Gain=inv_Lsource
  7 : Gain  Gain=Lsource
  8 : Gain  Gain=Csource
  9 : Gain  Gain=inv_Csource
  Demux1 : Demux  Outputs=2
  Demux2 : Demux  Outputs=2
  Id : Scope
  Iline_D_int : Integrator  UpperSaturationLimit=50  LowerSaturationLimit=-1000
  Iline_Q_int : Integrator  UpperSaturationLimit=50  LowerSaturationLimit=-1000
  Iq : Scope
  Mux1 : Mux  Inputs=2
  Mux2 : Mux  Inputs=2
  Product{1..2,7..8} (4 alike) : Product
  Sum1 : Sum  Inputs=|+---
  Sum14 : Sum  Inputs=|+--
  Sum15 : Sum  Inputs=|++-
  Sum8 : Sum  Inputs=|+-+-
  Vcd : Scope  Commented=on
  Vcfd_int : Integrator  UpperSaturationLimit=50  LowerSaturationLimit=-1000
  Vcfq_int : Integrator  UpperSaturationLimit=50  LowerSaturationLimit=-1000
  Vcq : Scope
  Iline_DQ : Outport  VectorParamsAs1DForOutWhenUnconnected=off
  Vpcc_DQ : Outport  Port=2  VectorParamsAs1DForOutWhenUnconnected=off
  wires:
  Mux2/1 -> Iline_DQ/1
  Iinv_DQ/1 -> Demux2/1
  Demux2/2 -> Sum14/1
  Demux2/1 -> Sum15/2
  [wL] -> Product2/1, Product1/1
  Product1/1 -> Sum1/3
  4/1 -> Iline_Q_int/1
  3/1 -> Sum1/4
  Product2/1 -> Sum8/3
  2/1 -> Sum8/4
  Sum8/1 -> 1/1
  Iline_Q_int/1 -> 3/1, Product2/2, Iq/1, [Iq], Mux2/2
  Iline_D_int/1 -> Mux2/1, 2/1, Id/1, Product1/2, [Id]
  1/1 -> Iline_D_int/1
  Sum1/1 -> 4/1
  [Vpcc_D] -> Sum8/1
  [Vpcc_Q] -> Sum1/1
  omega_ref/1 -> 8/1, 7/1
  7/1 -> [wL]
  9/1 -> Vcfd_int/1
  Sum14/1 -> 10/1
  [wcs] -> Product8/1, Product7/1
  [Id] -> Sum15/3
  Vcfq_int/1 -> Mux1/2, [Vpcc_Q], Product7/2, Vcq/1
  Product7/1 -> Sum15/1
  [Iq] -> Sum14/2
  10/1 -> Vcfq_int/1
  Sum15/1 -> 9/1
  Product8/1 -> Sum14/3
  8/1 -> [wcs]
  Vcfd_int/1 -> Product8/2, Mux1/1, [Vpcc_D], Vcd/1
  Mux1/1 -> Vpcc_DQ/1
  Demux1/1 -> Sum8/2
  Demux1/2 -> Sum1/2
  "VsDQ "/1 -> Demux1/1

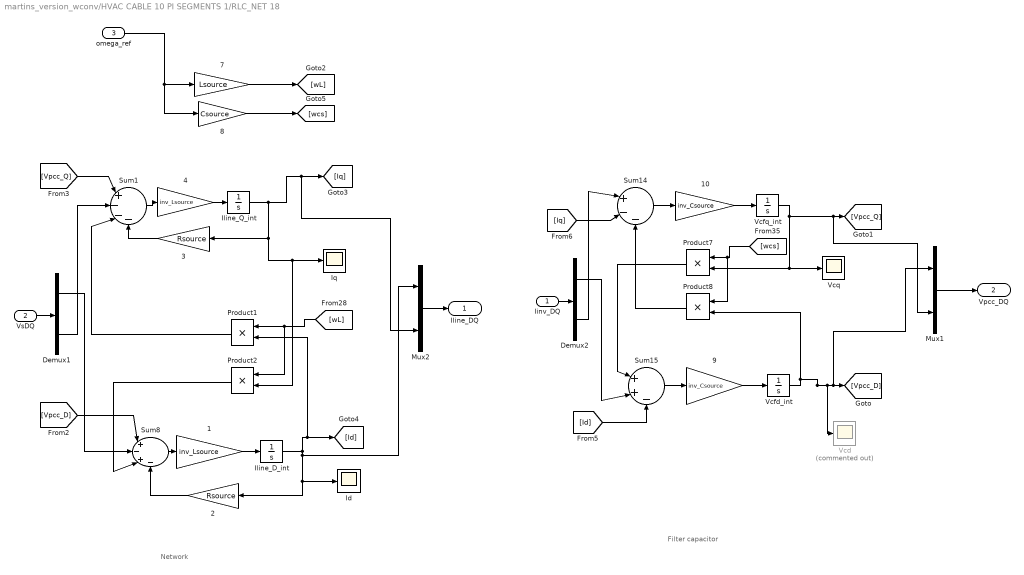
== system martins_version_wconv/HVAC CABLE 10 PI SEGMENTS 1/RLC_NET 18 ==
  note: Network
  note: Filter capacitor
  Iinv_DQ : Inport
  "VsDQ " : Inport  Port=2
  omega_ref : Inport  Port=3
  1 : Gain  Gain=inv_Lsource
  10 : Gain  Gain=inv_Csource
  2 : Gain  Gain=Rsource
  3 : Gain  Gain=Rsource
  4 : Gain  Gain=inv_Lsource
  7 : Gain  Gain=Lsource
  8 : Gain  Gain=Csource
  9 : Gain  Gain=inv_Csource
  Demux1 : Demux  Outputs=2
  Demux2 : Demux  Outputs=2
  Id : Scope
  Iline_D_int : Integrator  UpperSaturationLimit=50  LowerSaturationLimit=-1000
  Iline_Q_int : Integrator  UpperSaturationLimit=50  LowerSaturationLimit=-1000
  Iq : Scope
  Mux1 : Mux  Inputs=2
  Mux2 : Mux  Inputs=2
  Product{1..2,7..8} (4 alike) : Product
  Sum1 : Sum  Inputs=|+---
  Sum14 : Sum  Inputs=|+--
  Sum15 : Sum  Inputs=|++-
  Sum8 : Sum  Inputs=|+-+-
  Vcd : Scope  Commented=on
  Vcfd_int : Integrator  UpperSaturationLimit=50  LowerSaturationLimit=-1000
  Vcfq_int : Integrator  UpperSaturationLimit=50  LowerSaturationLimit=-1000
  Vcq : Scope
  Iline_DQ : Outport  VectorParamsAs1DForOutWhenUnconnected=off
  Vpcc_DQ : Outport  Port=2  VectorParamsAs1DForOutWhenUnconnected=off
  wires:
  Mux2/1 -> Iline_DQ/1
  Iinv_DQ/1 -> Demux2/1
  Demux2/2 -> Sum14/1
  Demux2/1 -> Sum15/2
  [wL] -> Product2/1, Product1/1
  Product1/1 -> Sum1/3
  4/1 -> Iline_Q_int/1
  3/1 -> Sum1/4
  Product2/1 -> Sum8/3
  2/1 -> Sum8/4
  Sum8/1 -> 1/1
  Iline_Q_int/1 -> 3/1, Product2/2, Iq/1, [Iq], Mux2/2
  Iline_D_int/1 -> Mux2/1, 2/1, Id/1, Product1/2, [Id]
  1/1 -> Iline_D_int/1
  Sum1/1 -> 4/1
  [Vpcc_D] -> Sum8/1
  [Vpcc_Q] -> Sum1/1
  omega_ref/1 -> 8/1, 7/1
  7/1 -> [wL]
  9/1 -> Vcfd_int/1
  Sum14/1 -> 10/1
  [wcs] -> Product8/1, Product7/1
  [Id] -> Sum15/3
  Vcfq_int/1 -> Mux1/2, [Vpcc_Q], Product7/2, Vcq/1
  Product7/1 -> Sum15/1
  [Iq] -> Sum14/2
  10/1 -> Vcfq_int/1
  Sum15/1 -> 9/1
  Product8/1 -> Sum14/3
  8/1 -> [wcs]
  Vcfd_int/1 -> Product8/2, Mux1/1, [Vpcc_D], Vcd/1
  Mux1/1 -> Vpcc_DQ/1
  Demux1/1 -> Sum8/2
  Demux1/2 -> Sum1/2
  "VsDQ "/1 -> Demux1/1

== system martins_version_wconv/HVAC CABLE 10 PI SEGMENTS 1/RLC_NET 19 ==
  note: Filter capacitor
  note: Network
  Iinv_DQ : Inport
  "VsDQ " : Inport  Port=2
  omega_ref : Inport  Port=3
  1 : Gain  Gain=inv_Lsource
  10 : Gain  Gain=inv_Csource
  2 : Gain  Gain=Rsource
  3 : Gain  Gain=Rsource
  4 : Gain  Gain=inv_Lsource
  7 : Gain  Gain=Lsource
  8 : Gain  Gain=Csource
  9 : Gain  Gain=inv_Csource
  Demux1 : Demux  Outputs=2
  Demux2 : Demux  Outputs=2
  Id : Scope
  Iline_D_int : Integrator  UpperSaturationLimit=50  LowerSaturationLimit=-1000
  Iline_Q_int : Integrator  UpperSaturationLimit=50  LowerSaturationLimit=-1000
  Iq : Scope
  Mux1 : Mux  Inputs=2
  Mux2 : Mux  Inputs=2
  Product{1..2,7..8} (4 alike) : Product
  Sum1 : Sum  Inputs=|+---
  Sum14 : Sum  Inputs=|+--
  Sum15 : Sum  Inputs=|++-
  Sum8 : Sum  Inputs=|+-+-
  Vcd : Scope  Commented=on
  Vcfd_int : Integrator  UpperSaturationLimit=50  LowerSaturationLimit=-1000
  Vcfq_int : Integrator  UpperSaturationLimit=50  LowerSaturationLimit=-1000
  Vcq : Scope
  Iline_DQ : Outport  VectorParamsAs1DForOutWhenUnconnected=off
  Vpcc_DQ : Outport  Port=2  VectorParamsAs1DForOutWhenUnconnected=off
  wires:
  "VsDQ "/1 -> Demux1/1
  Demux1/2 -> Sum1/2
  Demux1/1 -> Sum8/2
  Mux1/1 -> Vpcc_DQ/1
  Vcfd_int/1 -> Vcd/1, [Vpcc_D], Mux1/1, Product8/2
  8/1 -> [wcs]
  Product8/1 -> Sum14/3
  Sum15/1 -> 9/1
  10/1 -> Vcfq_int/1
  [Iq] -> Sum14/2
  Product7/1 -> Sum15/1
  Vcfq_int/1 -> Vcq/1, Product7/2, [Vpcc_Q], Mux1/2
  [Id] -> Sum15/3
  [wcs] -> Product7/1, Product8/1
  Sum14/1 -> 10/1
  9/1 -> Vcfd_int/1
  7/1 -> [wL]
  omega_ref/1 -> 7/1, 8/1
  [Vpcc_Q] -> Sum1/1
  [Vpcc_D] -> Sum8/1
  Sum1/1 -> 4/1
  1/1 -> Iline_D_int/1
  Iline_D_int/1 -> [Id], Product1/2, Id/1, 2/1, Mux2/1
  Iline_Q_int/1 -> Mux2/2, [Iq], Iq/1, Product2/2, 3/1
  Sum8/1 -> 1/1
  2/1 -> Sum8/4
  Product2/1 -> Sum8/3
  3/1 -> Sum1/4
  4/1 -> Iline_Q_int/1
  Product1/1 -> Sum1/3
  [wL] -> Product1/1, Product2/1
  Demux2/1 -> Sum15/2
  Demux2/2 -> Sum14/1
  Iinv_DQ/1 -> Demux2/1
  Mux2/1 -> Iline_DQ/1

== system martins_version_wconv/HVAC CABLE 10 PI SEGMENTS 1/RLC_NET 20 ==
  note: Network
  note: Filter capacitor
  Iinv_DQ : Inport
  "VsDQ " : Inport  Port=2
  omega_ref : Inport  Port=3
  1 : Gain  Gain=inv_Lsource
  10 : Gain  Gain=inv_Csource
  2 : Gain  Gain=Rsource
  3 : Gain  Gain=Rsource
  4 : Gain  Gain=inv_Lsource
  7 : Gain  Gain=Lsource
  8 : Gain  Gain=Csource
  9 : Gain  Gain=inv_Csource
  Demux1 : Demux  Outputs=2
  Demux2 : Demux  Outputs=2
  Id : Scope
  Iline_D_int : Integrator  UpperSaturationLimit=50  LowerSaturationLimit=-1000
  Iline_Q_int : Integrator  UpperSaturationLimit=50  LowerSaturationLimit=-1000
  Iq : Scope
  Mux1 : Mux  Inputs=2
  Mux2 : Mux  Inputs=2
  Product{1..2,7..8} (4 alike) : Product
  Sum1 : Sum  Inputs=|+---
  Sum14 : Sum  Inputs=|+--
  Sum15 : Sum  Inputs=|++-
  Sum8 : Sum  Inputs=|+-+-
  Vcd : Scope  Commented=on
  Vcfd_int : Integrator  UpperSaturationLimit=50  LowerSaturationLimit=-1000
  Vcfq_int : Integrator  UpperSaturationLimit=50  LowerSaturationLimit=-1000
  Vcq : Scope
  Iline_DQ : Outport  VectorParamsAs1DForOutWhenUnconnected=off
  Vpcc_DQ : Outport  Port=2  VectorParamsAs1DForOutWhenUnconnected=off
  wires:
  Mux2/1 -> Iline_DQ/1
  Iinv_DQ/1 -> Demux2/1
  Demux2/2 -> Sum14/1
  Demux2/1 -> Sum15/2
  [wL] -> Product2/1, Product1/1
  Product1/1 -> Sum1/3
  4/1 -> Iline_Q_int/1
  3/1 -> Sum1/4
  Product2/1 -> Sum8/3
  2/1 -> Sum8/4
  Sum8/1 -> 1/1
  Iline_Q_int/1 -> 3/1, Product2/2, Iq/1, [Iq], Mux2/2
  Iline_D_int/1 -> Mux2/1, 2/1, Id/1, Product1/2, [Id]
  1/1 -> Iline_D_int/1
  Sum1/1 -> 4/1
  [Vpcc_D] -> Sum8/1
  [Vpcc_Q] -> Sum1/1
  omega_ref/1 -> 8/1, 7/1
  7/1 -> [wL]
  9/1 -> Vcfd_int/1
  Sum14/1 -> 10/1
  [wcs] -> Product8/1, Product7/1
  [Id] -> Sum15/3
  Vcfq_int/1 -> Mux1/2, [Vpcc_Q], Product7/2, Vcq/1
  Product7/1 -> Sum15/1
  [Iq] -> Sum14/2
  10/1 -> Vcfq_int/1
  Sum15/1 -> 9/1
  Product8/1 -> Sum14/3
  8/1 -> [wcs]
  Vcfd_int/1 -> Product8/2, Mux1/1, [Vpcc_D], Vcd/1
  Mux1/1 -> Vpcc_DQ/1
  Demux1/1 -> Sum8/2
  Demux1/2 -> Sum1/2
  "VsDQ "/1 -> Demux1/1

== system martins_version_wconv/HVAC CABLE 10 PI SEGMENTS 1/RLV_NET 1 ==
  note: Network
  note: VIRTUAL RESITANCE
  Vpcc_DQ : Inport
  omega_ref : Inport  Port=2
  1 : Gain  Gain=inv_Lsource
  2 : Gain  Gain=Rsource
  3 : Gain  Gain=Rsource
  4 : Gain  Gain=inv_Lsource
  7 : Gain  Gain=Lsource
  Demux2 : Demux  Outputs=2
  Id : Scope
  Iline_D_int : Integrator  UpperSaturationLimit=50  LowerSaturationLimit=-1000
  Iline_Q_int : Integrator  UpperSaturationLimit=50  LowerSaturationLimit=-1000
  Iq : Scope
  Mux1 : Mux  Inputs=2
  Mux4 : Mux  Inputs=2
  Product1 : Product
  Product2 : Product
  Sum1 : Sum  Inputs=|+--
  Sum8 : Sum  Inputs=|++-
  Iline_DQ : Outport  VectorParamsAs1DForOutWhenUnconnected=off
  wires:
  Mux1/1 -> Iline_DQ/1
  Product2/1 -> Sum8/2
  3/1 -> Sum1/2
  7/1 -> [wL]
  [omega_ref] -> ?
  [Vpcc_Q] -> Sum1/1
  [Vpcc_D] -> Sum8/1
  Demux2/1 -> Mux4/1, [Vpcc_D]
  Demux2/2 -> Mux4/2, [Vpcc_Q]
  Sum1/1 -> 4/1
  1/1 -> Iline_D_int/1
  Iline_D_int/1 -> Product1/2, Id/1, 2/1, Mux1/1
  Iline_Q_int/1 -> Mux1/2, Iq/1, Product2/2, 3/1
  Sum8/1 -> 1/1
  2/1 -> Sum8/3
  4/1 -> Iline_Q_int/1
  Product1/1 -> Sum1/3
  [wL] -> Product1/1, Product2/1
  Vpcc_DQ/1 -> Demux2/1
  omega_ref/1 -> 7/1

== system martins_version_wconv/HVAC CABLE 10 PI SEGMENTS 1/RLV_NET 2 ==
  note: VIRTUAL RESITANCE
  note: Network
  Vpcc_DQ : Inport
  omega_ref : Inport  Port=2
  1 : Gain  Gain=inv_Lsource
  2 : Gain  Gain=Rsource
  3 : Gain  Gain=Rsource
  4 : Gain  Gain=inv_Lsource
  7 : Gain  Gain=Lsource
  Demux2 : Demux  Outputs=2
  Id : Scope
  Iline_D_int : Integrator  UpperSaturationLimit=50  LowerSaturationLimit=-1000
  Iline_Q_int : Integrator  UpperSaturationLimit=50  LowerSaturationLimit=-1000
  Iq : Scope
  Mux1 : Mux  Inputs=2
  Mux4 : Mux  Inputs=2
  Product1 : Product
  Product2 : Product
  Sum1 : Sum  Inputs=|+--
  Sum8 : Sum  Inputs=|++-
  Iline_DQ : Outport  VectorParamsAs1DForOutWhenUnconnected=off
  wires:
  omega_ref/1 -> 7/1
  Vpcc_DQ/1 -> Demux2/1
  [wL] -> Product2/1, Product1/1
  Product1/1 -> Sum1/3
  4/1 -> Iline_Q_int/1
  2/1 -> Sum8/3
  Sum8/1 -> 1/1
  Iline_Q_int/1 -> 3/1, Product2/2, Iq/1, Mux1/2
  Iline_D_int/1 -> Mux1/1, 2/1, Id/1, Product1/2
  1/1 -> Iline_D_int/1
  Sum1/1 -> 4/1
  Demux2/2 -> [Vpcc_Q], Mux4/2
  Demux2/1 -> [Vpcc_D], Mux4/1
  [Vpcc_D] -> Sum8/1
  [Vpcc_Q] -> Sum1/1
  [omega_ref] -> ?
  7/1 -> [wL]
  3/1 -> Sum1/2
  Product2/1 -> Sum8/2
  Mux1/1 -> Iline_DQ/1

== system martins_version_wconv/GFC_WT/Active power loop//Electromechanical/Subsystem ==
  In1 : Inport
  Gain1 : Gain  Gain=KI_LL
  Gain2 : Gain  Commented=on  Gain=KP_LL
  Integrator : Integrator
  PID Controller : slpidlib/PID Controller  Controller=P  Form=Parallel  TimeDomain=Continuous-time  UseExternalTs=off  SampleTime=-1  IntegratorMethod=Forward Euler  FilterMethod=Forward Euler  ControllerParametersSource=internal  P=KP_LL  I=1  UseKiTs=off  D=0  N=100  UseFilter=on  TunerSelectOption=Transfer Function Based (PID Tuner App)  InitialConditionSource=internal  InitialConditionForIntegrator=0  InitialConditionForFilter=0  DifferentiatorICPrevScaledInput=0  ExternalReset=none  TrackingMode=off  Kt=1  LimitOutput=off  SatLimitsSource=internal  UpperSaturationLimit=inf  LowerSaturationLimit=-inf  LinearizeAsGain=on  AntiWindupMode=none  Kb=1  LimitIntegrator=off  UpperIntegratorSaturationLimit=inf  LowerIntegratorSaturationLimit=-inf  POutMin=[]  POutMax=[]  IOutMin=[]  IOutMax=[]  DOutMin=[]  DOutMax=[]  NOutMin=[]  NOutMax=[]  SumOutMin=[]  SumOutMax=[]  SaturationOutMin=[]  SaturationOutMax=[]  PParamMin=[]  PParamMax=[]  IParamMin=[]  IParamMax=[]  DParamMin=[]  DParamMax=[]  NParamMin=[]  NParamMax=[]  KbParamMin=[]  KbParamMax=[]  KtParamMin=[]  KtParamMax=[]  KbOutMin=[]  KbOutMax=[]  KtOutMin=[]  KtOutMax=[]  IntegratorOutMin=[]  IntegratorOutMax=[]  FilterOutMin=[]  FilterOutMax=[]  SumI1OutMin=[]  SumI1OutMax=[]  SumI2OutMin=[]  SumI2OutMax=[]  SumI3OutMin=[]  SumI3OutMax=[]  SumI4OutMin=[]  SumI4OutMax=[]  SumDOutMin=[]  SumDOutMax=[]  DifferentiatorOutMin=[]  DifferentiatorOutMax=[]  FilterDiffOutCoefMin=[]  FilterDiffOutCoefMax=[]  ReciprocalOutMin=[]  ReciprocalOutMax=[]  SumDenOutMin=[]  SumDenOutMax=[]  SumNumOutMin=[]  SumNumOutMax=[]  DivideOutMin=[]  DivideOutMax=[]  UdiffTsProdOutMin=[]  UdiffTsProdOutMax=[]  NTsProdOutMin=[]  NTsProdOutMax=[]  UintegralTsProdOutMin=[]  UintegralTsProdOutMax=[]  UngainTsProdOutMin=[]  UngainTsProdOutMax=[]  ClampingZeroOutDataTypeStr=Inherit: Inherit via back propagation  ClampingZeroOutMin=[]  ClampingZeroOutMax=[]  FilterDenConstantOutDataTypeStr=Inherit: Inherit via back propagation  FilterDenConstantOutMin=[]  FilterDenConstantOutMax=[]  PCopyOutDataTypeStr=Inherit: Inherit via back propagation  PCopyOutMin=[]  PCopyOutMax=[]  NCopyOutDataTypeStr=Inherit: Inherit via back propagation  NCopyOutMin=[]  NCopyOutMax=[]  IntegratorContinuousStateAttributes=''  IntegratorStateMustResolveToSignalObject=off  IntegratorRTWStateStorageClass=Auto  FilterContinuousStateAttributes=''  FilterStateMustResolveToSignalObject=off  FilterRTWStateStorageClass=Auto  ParallelPVariant=InternalParameters  IdealPVariant=Disabled  IVariant=Disabled  DVariant=Disabled  IntegratorVariant=Disabled  SatVariant=Disabled  AWVariant=Disabled  PCopyVariant=Disabled  TRVariant=Disabled  FdbkBlocksVariant=Forward  IdealPFdbkVariant=Disabled  SatFdbkVariant=Disabled  DerivativeFilterVariant=Disabled  NVariant=Disabled  NCopyVariant=Disabled_SignalSpec  FilterICVariant=Disabled  IntegratorICVariant=Disabled  ExternalResetVariant=Disabled  TRSumVariant=Passthrough  SumFdbkVariant=Disabled  SumVariant=Passthrough_P  TsampFilterVariant=InternalTs  TsampNgainVariant=Passthrough  TsampIntegralVariant=Disabled_SignalSpec  ExternalSaturationOutDataTypeStr=Inherit: Same as second input
  Sum1 : Sum  Inputs=|++
  Out1 : Outport
  wires:
  Sum1/1 -> Out1/1
  Gain1/1 -> Integrator/1
  In1/1 -> Gain1/1, PID Controller/1
  PID Controller/1 -> Sum1/1
  Integrator/1 -> Sum1/2

== system martins_version_wconv/GFC_WT/DC-link voltage controller/DC init ==
  second : Inport
  init : Inport  Port=2
  Clock : Clock
  Switch : Switch  Criteria=u2 > Threshold  Threshold=10  SaturateOnIntegerOverflow=off  InputSameDT=off
  "   " : Outport
  wires:
  second/1 -> Switch/1
  init/1 -> Switch/3
  Clock/1 -> Switch/2
  Switch/1 -> "   "/1

== system martins_version_wconv/GFC_WT/Subsystem/Current Control ==
  i_cv_ref : Inport
  v_o : Inport  Port=2
  i_o : Inport  Port=3
  i_cv : Inport  Port=4
  AD : Gain  Gain=-k_AD  SaturateOnIntegerOverflow=on  OutDataTypeStr=Inherit: Same as input  ParamDataTypeStr=Inherit: Same as input
  AD1 : Gain  Gain=-l_f*k_decouple  SaturateOnIntegerOverflow=on  OutDataTypeStr=Inherit: Same as input  ParamDataTypeStr=Inherit: Same as input
  AD2 : Gain  Gain=l_f*k_decouple  SaturateOnIntegerOverflow=on  OutDataTypeStr=Inherit: Same as input  ParamDataTypeStr=Inherit: Same as input
  Demux4 : Demux  Outputs=[vect vect]
  Display : Display
  Mux5 : Mux  Inputs=[vect vect]
  PI : Subsystem
  Product : Product
  Step : Step  SampleTime=0
  Sum : Sum  Inputs=|++
  Sum1 : Sum  Inputs=-+|  InputSameDT=on  SaturateOnIntegerOverflow=on  OutDataTypeStr=Inherit: Same as first input
  Sum4 : Sum  Inputs=++++  InputSameDT=on  SaturateOnIntegerOverflow=on  OutDataTypeStr=Inherit: Same as first input
  Sum5 : Sum  Inputs=|+-  InputSameDT=on  SaturateOnIntegerOverflow=on  OutDataTypeStr=Inherit: Same as first input
  decoupling : Gain  Gain=r_f  Multiplication=Matrix(K*u)
  decoupling1 : Gain  Commented=on  Gain=(r_f*eye(2)+[0,-1; 1,0])*l_f*k_decouple  Multiplication=Matrix(K*u)
  i_cv_ref_ : Scope
  i_cv_ref_1 : Scope
  v_ff : Gain  Gain=k_ffv  SaturateOnIntegerOverflow=on  OutDataTypeStr=Inherit: Same as input  ParamDataTypeStr=Inherit: Same as input
  v_ref_dq : Outport  VectorParamsAs1DForOutWhenUnconnected=off
  wires:
  v_o/1 -> v_ff/1
  v_ff/1 -> Sum4/1
  i_o/1 -> Sum5/1
  Sum5/1 -> AD/1
  Sum1/1 -> Product/2, i_cv_ref_1/1
  AD/1 -> Display/1, Sum4/2
  PI/1(pi_out) -> Sum4/4
  i_cv/1 -> decoupling/1, Sum5/2, Sum1/1, Demux4/1
  i_cv_ref/1 -> i_cv_ref_/1, Sum1/2
  Sum4/1 -> v_ref_dq/1
  Demux4/2 -> AD1/1
  Demux4/1 -> AD2/1
  AD1/1 -> Mux5/1
  AD2/1 -> Mux5/2
  Mux5/1 -> Sum/2
  decoupling/1 -> Sum/1
  Sum/1 -> Sum4/3
  Product/1 -> PI/1(i_cv_err)
  Step/1 -> Product/1

== system martins_version_wconv/GFC_WT/Subsystem/Current Limit Logic ==
  note: Circular Current limiter
  I_ref_unsat : Inport
  Abs1 : Abs
  Constant3 : Constant
  Constant4 : Constant  Value=1.2
  Demux6 : Demux  Outputs=2
  Demux7 : Demux  Outputs=[vect vect]
  Display3 : Display
  Divide : Product  Inputs=*/
  Divide1 : Product  Inputs=*/
  First-Order Filter1 : spsFirstOrderFilterLib/First-Order Filter  FilterType=Lowpass  Tc=0.002  Ts=0  Initialize=on  Vac_Init=[0, 0, 60]  Vdc_Init=0  PlotResponse=off  FreqRange="[0,  200,  1]"
  GreaterThan1 : RelationalOperator  Operator=>  OutDataTypeStr=boolean  RndMeth=Simplest  InputSameDT=off
  I_d_error2 : Scope  Commented=on
  I_d_error3 : Scope  Commented=on
  I_d_error5 : Scope  Commented=on
  Kip12 : Gain
  Kip13 : Gain  Gain=1/1.2
  Mux6 : Mux  Inputs=[vect vect]
  Real-Imag to Complex1 : RealImagToComplex
  Switch1 : Switch  Threshold=1  SaturateOnIntegerOverflow=off  InputSameDT=off
  Unit Delay2 : UnitDelay  InitialCondition=1  SampleTime=-1  HasFrameUpgradeWarning=on
  Vmd2 : Display
  I_ref_sat : Outport
  wires:
  First-Order Filter1/1 -> Demux6/1
  Kip12/1 -> Unit Delay2/1, Display3/1
  Divide/1 -> Mux6/1
  Switch1/1 -> I_d_error3/1, Kip12/1
  Constant4/1 -> GreaterThan1/2
  Kip13/1 -> Switch1/1
  Constant3/1 -> Switch1/3
  Demux7/1 -> Divide/1
  I_ref_unsat/1 -> First-Order Filter1/1, Vmd2/1, I_d_error5/1, Demux7/1
  Demux6/1 -> Real-Imag to Complex1/1
  GreaterThan1/1 -> Switch1/2
  Demux7/2 -> Divide1/1
  Real-Imag to Complex1/1 -> Abs1/1
  Unit Delay2/1 -> Divide/2, Divide1/2
  Abs1/1 -> GreaterThan1/1, I_d_error2/1, Kip13/1
  Demux6/2 -> Real-Imag to Complex1/2
  Divide1/1 -> Mux6/2
  Mux6/1 -> I_ref_sat/1

== system martins_version_wconv/GFC_WT/Subsystem/PLL>>grid2 ==
  note: inv ([  cos(wt)   sin(wt)
      |    -sin(wt)    cos(wt)   ])
  note: =
  note: [  al
      |     be  ]
  note: =
  note: [  al
      |     be  ]
  note: [ d
      |    q ]
  note: *
  note: [ d
      |    q ]
  note: [  cos(wt)   -sin(wt)
      |    sin(wt)    cos(wt)   ]
  note: *
  vgdq : Inport
  thetaPLL : Inport  Port=2
  Cos : Trigonometry  Operator=cos
  Demux1 : Demux  Outputs=2
  Display5 : Display
  Mux3 : Mux  Inputs=2
  Product{,1..3} (4 alike) : Product
  Sin : Trigonometry
  Sum : Sum  Inputs=+-
  Sum1 : Sum
  vgDQ : Outport  InitialOutput=[0,0]  VectorParamsAs1DForOutWhenUnconnected=off
  wires:
  vgdq/1 -> Demux1/1
  thetaPLL/1 -> Cos/1, Sin/1
  Sin/1 -> Product3/2, Product1/2
  Demux1/1 -> Product3/1, Product/1
  Cos/1 -> Product2/2, Product/2
  Product/1 -> Sum/1
  Demux1/2 -> Product2/1, Product1/1
  Product1/1 -> Sum/2
  Sum/1 -> Mux3/1
  Product2/1 -> Sum1/1
  Product3/1 -> Sum1/2
  Sum1/1 -> Mux3/2
  Mux3/1 -> Display5/1, vgDQ/1

== system martins_version_wconv/GFC_WT/Subsystem/RL filter ==
  note: Inverter side inductor
  In1 : Inport
  In2 : Inport  Port=2
  In3 : Inport  Port=3
  In4 : Inport  Port=4
  In5 : Inport  Port=5
  1 : Gain  Gain=r_f_si1
  2 : Gain  Gain=1/(l_f_si1)
  3 : Gain  Gain=r_f_si1
  4 : Gain  Gain=1/(l_f_si1)
  Id : Scope
  Id_int : Integrator  UpperSaturationLimit=50  LowerSaturationLimit=-1000
  Iq : Scope
  Iq_int : Integrator  UpperSaturationLimit=50  LowerSaturationLimit=-1000
  L value : Constant  Value=l_f_si1  SampleTime=-1
  Product : Product
  Product1 : Product
  Product2 : Product
  Sum1 : Sum  Inputs=|+---
  Sum8 : Sum  Inputs=|+-+-
  id1 : Display
  Out1 : Outport
  Out2 : Outport  Port=2
  wires:
  In5/1 -> Product/1
  Product/1 -> [wL], id1/1
  L value/1 -> Product/2
  In1/1 -> Sum1/2
  In3/1 -> Sum1/1
  In4/1 -> Sum8/2
  In2/1 -> Sum8/1
  Product2/1 -> Sum8/3
  Iq_int/1 -> Iq/1, Product2/2, 3/1, Out1/1
  4/1 -> Iq_int/1
  Sum8/1 -> 2/1
  2/1 -> Id_int/1
  Sum1/1 -> 4/1
  3/1 -> Sum1/4
  Product1/1 -> Sum1/3
  1/1 -> Sum8/4
  Id_int/1 -> Product1/2, Out2/1, Id/1, 1/1
  [wL] -> Product1/1, Product2/1

== system martins_version_wconv/GFC_WT/Subsystem/Virtual Admittance1 ==
  delvdq : Inport
  omega_PLL : Inport  Port=2
  5 : Gain  Gain=R_Virt
  Demux2 : Demux  Outputs=[vect vect]
  Divide : Product  Inputs=*/
  Divide1 : Product  Inputs=*/
  L value : Constant  Value=L_Virt  SampleTime=-1
  L value1 : Constant  Value=R_Virt*ones(vect,1)  SampleTime=-1
  L value2 : Constant  SampleTime=-1
  Mux4 : Mux  Inputs=[vect vect]
  Product{,1..4} (5 alike) : Product
  Square : Math  Operator=square
  Square1 : Math  Operator=square
  Sum : Sum  Inputs=|++
  Sum1 : Sum  Inputs=|++
  Sum2 : Sum  Inputs=|+-
  id{1..4} (4 alike) : Display
  Idqref : Outport
  wires:
  Mux4/1 -> id3/1, Idqref/1
  delvdq/1 -> id4/1, Demux2/1
  Product/1 -> Divide1/1, id1/1, Square1/1
  omega_PLL/1 -> Product/1
  L value/1 -> Product/2
  L value1/1 -> Square/1
  Square1/1 -> Sum/1
  Square/1 -> Sum/2
  Sum/1 -> id2/1, Divide1/2, Divide/2
  L value2/1 -> Divide/1
  Divide/1 -> 5/1
  5/1 -> Product3/1, Product1/1
  Demux2/1 -> Product4/1, Product1/2
  Divide1/1 -> Product4/2, Product2/1
  Demux2/2 -> Product2/2, Product3/2
  Product2/1 -> Sum1/1
  Product1/1 -> Sum1/2
  Sum1/1 -> Mux4/1
  Product3/1 -> Sum2/1
  Sum2/1 -> Mux4/2
  Product4/1 -> Sum2/2

== system martins_version_wconv/GFC_WT/Subsystem/Current Control/PI ==
  i_cv_err : Inport
  Demux : Demux  Outputs=[vect vect]
  Idreg : Subsystem
  Idreg1 : Subsystem
  Mux1 : Mux  Inputs=[vect vect]
  pi_out : Outport
  wires:
  Demux/2 -> Idreg1/1(In1)
  Idreg/1(W) -> Mux1/1
  Idreg1/1(W) -> Mux1/2
  Mux1/1 -> pi_out/1
  i_cv_err/1 -> Demux/1
  Demux/1 -> Idreg/1(In1)

== system martins_version_wconv/GFC_WT/Subsystem/Current Control/PI/Idreg ==
  In1 : Inport
  Integrator : Integrator
  Ppart : Gain  Gain=k_pc  SaturateOnIntegerOverflow=on  OutDataTypeStr=Inherit: Same as input  ParamDataTypeStr=Inherit: Same as input
  Ppart1 : Gain  Gain=k_ic  SaturateOnIntegerOverflow=on  OutDataTypeStr=Inherit: Same as input  ParamDataTypeStr=Inherit: Same as input
  Sum5 : Sum  Inputs=|++  InputSameDT=on  SaturateOnIntegerOverflow=on  OutDataTypeStr=Inherit: Same as first input
  W : Outport
  wires:
  Sum5/1 -> W/1  "W"
  Ppart/1 -> Sum5/1
  In1/1 -> Ppart1/1, Ppart/1
  Ppart1/1 -> Integrator/1
  Integrator/1 -> Sum5/2

== system martins_version_wconv/GFC_WT/Subsystem/Current Control/PI/Idreg1 ==
  In1 : Inport
  Integrator : Integrator
  Ppart : Gain  Gain=k_pc  SaturateOnIntegerOverflow=on  OutDataTypeStr=Inherit: Same as input  ParamDataTypeStr=Inherit: Same as input
  Ppart1 : Gain  Gain=k_ic  SaturateOnIntegerOverflow=on  OutDataTypeStr=Inherit: Same as input  ParamDataTypeStr=Inherit: Same as input
  Sum5 : Sum  Inputs=|++  InputSameDT=on  SaturateOnIntegerOverflow=on  OutDataTypeStr=Inherit: Same as first input
  W : Outport
  wires:
  Integrator/1 -> Sum5/2
  Ppart1/1 -> Integrator/1
  In1/1 -> Ppart/1, Ppart1/1
  Ppart/1 -> Sum5/1
  Sum5/1 -> W/1  "W"
